simulink model "testMdlVehicle"  (R2023a)
settings: Solver=VariableStepAuto  StartTime=0.0  StopTime=20  RelTol=1e-3
values from neighbouring files (symbols this model uses):
  vehicleObject = vehicle.sportSedan    [testVehicle.m]
undefined symbols (not defined in the file or in its folder): FrontLeft, FrontRight, RearLeft, RearRight
settings Model: Creator=grouleau  LastModifiedBy=grouleau
settings DataIOCC: DatasetSignalFormat=timetable

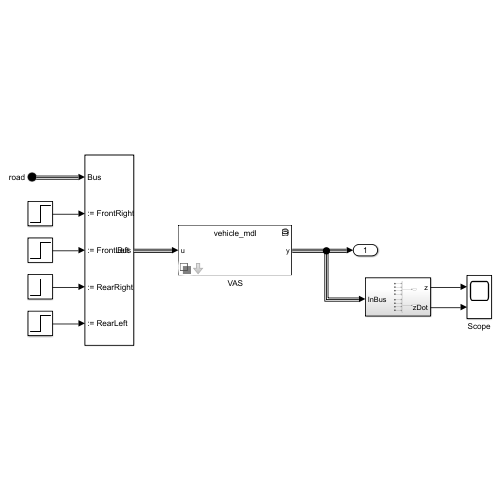
[thumbnail: Simulink's stored preview of the top-level diagram]
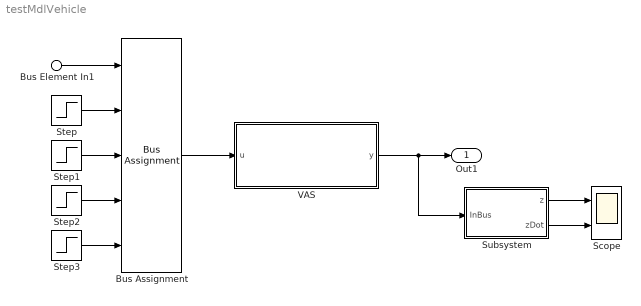
== system testMdlVehicle ==
  Bus Element In1 : Inport  PortName=road
  Bus Assignment : BusAssignment  AssignedSignals=FrontRight,FrontLeft,RearRight,RearLeft
  Scope : Scope  NumInputPorts=2
  Step : Step  Time=2  After=0.1  SampleTime=0
  Step1 : Step  Time=6  After=0.1  SampleTime=0
  Step2 : Step  Time=10  After=0.1  SampleTime=0
  Step3 : Step  Time=14  After=0.1  SampleTime=0
  Subsystem : Subsystem
  VAS : Subsystem  Variant=on  VariantChoicesSpecifier=obj.getVariantChoices()  VariantControlMode=label  LabelModeActiveChoice=vehicle_mdl  mask{obj=vehicleObject}
      mask prompts: obj "Part Object"
  Out1 : Outport
  wires:
  VAS/1(y) -> Subsystem/1(InBus), Out1/1
  Bus Element In1/1 -> Bus Assignment/1
  Step/1 -> Bus Assignment/2
  Bus Assignment/1 -> VAS/1(u)
  Step1/1 -> Bus Assignment/3
  Step2/1 -> Bus Assignment/4
  Step3/1 -> Bus Assignment/5
  Subsystem/1(z) -> Scope/1
  Subsystem/2(zDot) -> Scope/2

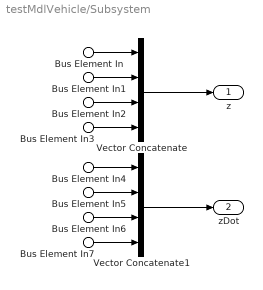
== system testMdlVehicle/Subsystem ==
  Bus Element In : Inport  PortName=InBus  Element=FrontLeft.z
  Bus Element In4 : Inport  PortName=InBus  Element=FrontLeft.zDot
  Bus Element In1 : Inport  PortName=InBus  Element=FrontRight.z
  Bus Element In5 : Inport  PortName=InBus  Element=FrontRight.zDot
  Bus Element In2 : Inport  PortName=InBus  Element=RearLeft.z
  Bus Element In6 : Inport  PortName=InBus  Element=RearLeft.zDot
  Bus Element In3 : Inport  PortName=InBus  Element=RearRight.z
  Bus Element In7 : Inport  PortName=InBus  Element=RearRight.zDot
  Vector Concatenate : Concatenate  NumInputs=4
  Vector Concatenate1 : Concatenate  NumInputs=4
  z : Outport
  zDot : Outport  Port=2
  wires:
  Bus Element In/1 -> Vector Concatenate/1
  Bus Element In1/1 -> Vector Concatenate/2
  Bus Element In2/1 -> Vector Concatenate/3
  Bus Element In3/1 -> Vector Concatenate/4
  Bus Element In4/1 -> Vector Concatenate1/1
  Bus Element In5/1 -> Vector Concatenate1/2
  Bus Element In6/1 -> Vector Concatenate1/3
  Bus Element In7/1 -> Vector Concatenate1/4
  Vector Concatenate/1 -> z/1
  Vector Concatenate1/1 -> zDot/1

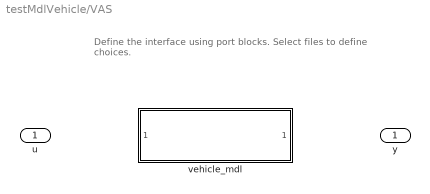
== system testMdlVehicle/VAS ==
  note: Define the interface using port blocks.
      | Select files to define choices.
  u : Inport
  vehicle_mdl : Subsystem  VariantControl=vehicle_mdl  ReferencedSubsystem=vehicle_mdl  obj=obj
  y : Outport
